simulink model "pe_estim_ami"  (Simulink 8.7)
settings: Solver=FixedStepDiscrete  SolverMode=SingleTasking  StartTime=0.0  StopTime=5000e-3  FixedStep=1/100000  RelTol=1e-3  AbsTol=1e-6
libraries: commchan3 x1, commsink2 x1, dspsrcs4 x1
settings Model: Creator=amoura  LastModifiedBy=Artur Moura
settings DataIOCC: LimitDataPoints=off  SignalLoggingSaveFormat=ModelDataLogs  SignalLoggingName=sigsOut
settings OptimizationCC: BooleanDataType=off  ExpressionDepthLimit=2147483647  InitFltsAndDblsToZero=on
settings DebuggingCC: SaveWithParameterizedLinksMsg=none  SignalResolutionControl=TryResolveAllWithWarning  MultiTaskDSMMsg=warning  MultiTaskCondExecSysMsg=none  FcnCallInpInsideContextMsg=UseLocalSettings  StateNameClashWarn=warning
settings HardwareCC: TargetUnknown=on
settings RTWCC: TemplateMakefile=grt_unix.tmf
settings GRTTargetCC: TargetFcnLib=ansi_tfl_tmw.mat  ModelReferenceCompliant=off  CombineOutputUpdateFcns=off  MatFileLogging=off  GRTInterface=on

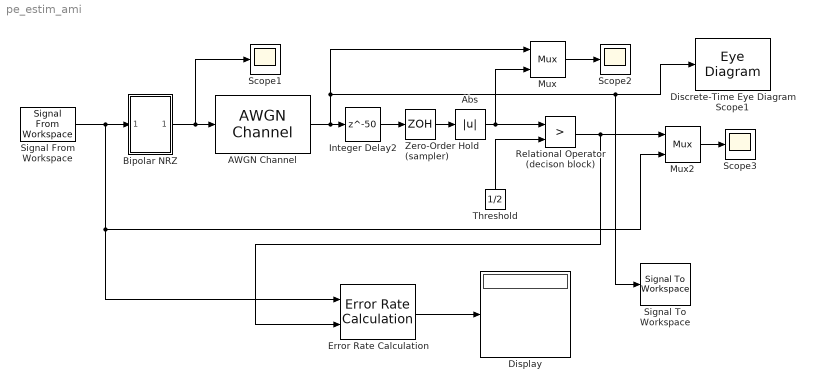
== system pe_estim_ami ==
  AWGN Channel : commchan3/AWGN Channel  InputProcessing=Columns as channels (frame based)  seed=67  noiseMode=Variance from mask  EbNodB=10  EsNodB=10  SNRdB=10  bitsPerSym=1  Ps=1  Tsym=1  variance=0.05
  Abs : Abs
  Bipolar NRZ : Subsystem  mask(Bipolar NRZ (AMI)){Ts=1/1000}
      mask prompts: Ts "Sample time (sec):"
      mask help:
      | This block encodes a unipolar NRZ signal into the bpolar NRZ
      | (non-return-to-zero) line code
      |
      | The output values are alternately +1 and -1 for nonzero  a nonzero input and  zero otherwise.
      mask Help:
      | This block encodes a unipolar NRZ signal into the bpolar NRZ
      | (non-return-to-zero) line code
      | 
      | The output values are alternately +1 and -1 for nonzero  a nonzero input and  zero otherwise.
      mask Display: disp('Bipolar\nNRZ\n(AMI)')
  Discrete-Time Eye Diagram Scope1 : EyeDiagram  Tag=EyeDiagram
  Display : Display
  Error Rate Calculation : commsink2/Error Rate Calculation  N=1  st_delay=1  cp_mode=Entire frame  subframe=[]  PMode=Port  WsName=ErrorVec  RsMode2=off  stop=off  numErr=100  maxBits=1e6
  Integer Delay2 : Delay  DelayLength=50  InputProcessing=Inherited  SampleTime=1/100000
  Mux : Mux  Inputs=2
  Mux2 : Mux  Inputs=2
  Relational Operator (decison block) : RelationalOperator  Operator=>  InputSameDT=on
  Scope1 : Scope
  Scope2 : Scope
  Scope3 : Scope
  Signal From Workspace : dspsrcs4/Signal From Workspace  X=randi([0,1],10000,1)  Ts=1/1000  nsamps=1  OutputAfterFinalValue=Cyclic repetition  ignoreOrWarnInputAndFrameLengths=off  OutputFrames=on
  Signal To Workspace : SignalToWorkspace  VariableName=simout
      settings: CopyFcn=dspblkcopystw(gcbh);
  Threshold : Constant  Value=1/2
  Zero-Order Hold (sampler) : ZeroOrderHold  SampleTime=1/1000
  wires:
  Mux2/1 -> Scope3/1
  Relational Operator (decison block)/1 -> Mux2/1, Error Rate Calculation/2
  Zero-Order Hold (sampler)/1 -> Abs/1
  Bipolar NRZ/1(Out1) -> Scope1/1, AWGN Channel/1
  Signal From Workspace/1 -> Mux2/2, Error Rate Calculation/1, Bipolar NRZ/1(In1)
  Error Rate Calculation/1 -> Display/1
  Mux/1 -> Scope2/1
  Threshold/1 -> Relational Operator (decison block)/2
  AWGN Channel/1 -> Mux/1, Discrete-Time Eye Diagram Scope1/1, Signal To Workspace/1, Integer Delay2/1
  Abs/1 -> Mux/2, Relational Operator (decison block)/1
  Integer Delay2/1 -> Zero-Order Hold (sampler)/1

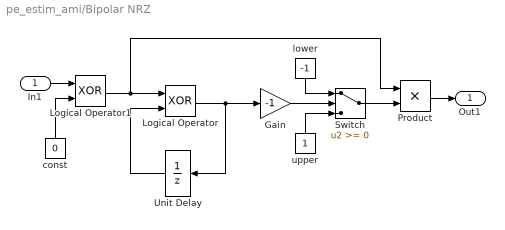
== system pe_estim_ami/Bipolar NRZ ==
  In1 : Inport
  Gain : Gain  Gain=-1  SaturateOnIntegerOverflow=on  OutDataTypeStr=Inherit: Same as input  ParamDataTypeStr=Inherit: Same as input
  Logical Operator : Logic  Operator=XOR
  Logical Operator1 : Logic  Operator=XOR
  Product : Product  SaturateOnIntegerOverflow=on  InputSameDT=on  OutDataTypeStr=Inherit: Same as first input
  Switch : Switch  SaturateOnIntegerOverflow=on  InputSameDT=on
  Unit Delay : UnitDelay  SampleTime=Ts
  const : Constant  Value=0
  lower : Constant  Value=-1
  upper : Constant
  Out1 : Outport
  wires:
  Unit Delay/1 -> Logical Operator/2
  Logical Operator/1 -> Gain/1, Unit Delay/1
  Gain/1 -> Switch/2
  upper/1 -> Switch/3
  lower/1 -> Switch/1
  const/1 -> Logical Operator1/2
  Switch/1 -> Product/2
  Logical Operator1/1 -> Logical Operator/1, Product/1
  In1/1 -> Logical Operator1/1
  Product/1 -> Out1/1
